simulink model "SolarPVMPPTBoost"  (R2025a)
settings: Solver=ode23t  StartTime=0.0  StopTime=t_sim2(end)  MaxStep=1/(10*solarPlant.converterSwitchingFrequency)  RelTol=1e-3  AbsTol=1e-3
PreLoadFcn:
  | run('SolarPVMPPTBoostData');
undefined symbols (not defined in the file or in its folder): boostController, dcVoltage, sensor, solarPanel, solarPlant
libraries: fl_lib x12, nesl_utility x10, simulink x6, ee_lib x3, batteryecm_lib x2, eePwmGenerator x2, simulink_extras x1
(part 1 of 2)
Description:
  | Solar PV System with MPPT Using Boost Converter
  | 
  | %
settings Model: Creator=The MathWorks, Inc.  LastModifiedBy=LaptopHP
settings SolverCC: AutoScaleAbsTol=off  AlgebraicLoopSolver=TrustRegion  MaxZcPerStep=1.0
settings DataIOCC: SaveOutput=off  DSMLogging=off  SaveTime=off  ReturnWorkspaceOutputs=off  SignalLoggingName=SolarPVMPPTBoost_logDB
settings OptimizationCC: ReuseModelBlockBuffer=off
settings DebuggingCC: UnconnectedInputMsg=warning  UnconnectedOutputMsg=warning  UnconnectedLineMsg=warning  SymbolicDimsDataTypeCodeGenerationDiagnostic=none
settings ModelReferenceCC: EnableRefExpFcnMdlSchedulingChecks=on
settings SFSimCC: CustomCodeUndefinedFunction=UseInterfaceOnly
settings RTWCC: GPUComputeCapability=3.5  DLArmComputeVersion=19.05
settings SimscapeCC: SimscapeLogType=all  SimscapeLogSimulationStatistics=on  SimscapeLogName=simlog_SolarPVMPPTBoost  SimscapeLogDataHistory=10000.0

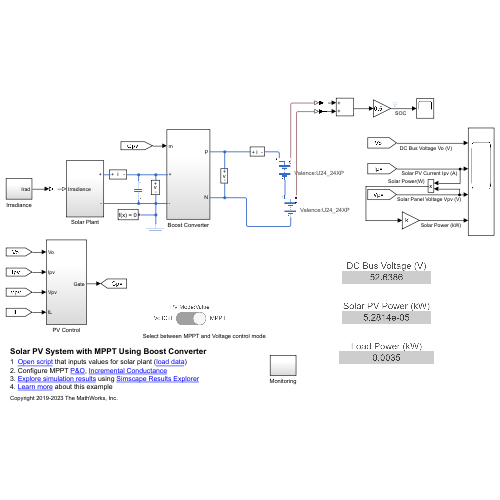
[thumbnail: Simulink's stored preview of the top-level diagram]
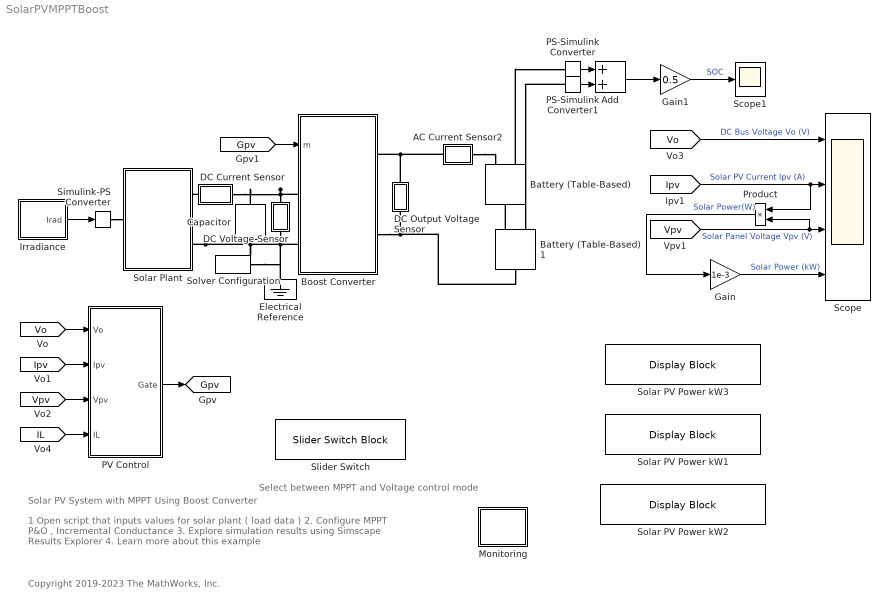
== system SolarPVMPPTBoost ==
  note: Select between MPPT and Voltage control mode
  note: Solar PV System with MPPT Using Boost Converter
  note: 1 Open script that inputs values for solar plant ( load data )
      | 2. Configure MPPT P&O , Incremental Conductance
      | 3. Explore simulation results using Simscape Results Explorer
      | 4. Learn more about this example
  note: Copyright 2019-2023 The MathWorks, Inc.
  AC Current Sensor2 : Subsystem
      mask Display: disp('i');
  Add : Sum
  Battery (Table-Based) : batteryecm_lib/Battery (Table-Based)  PartSpecification="{\"CollectionId\":\"SimscapeBatteryShared\",\"CollectionVersion\":\"1.0.0\",\"DatasetId\":\"Valence|U24_24XP|simscape.battery.batteryTableBased\",\"DisplayName\":\"Valence:U24_24XP\"}"  SOC_vec=[0 0.01 0.02 0.03 0.04 0.05 0.06 0.07 0.08 0.09 0.1 0.11 0.12 0.13 0.14 0.15 0.16 0.17 0.18 0.19 0.2 0.21 0.22 0.23 0.24 0.25 0.26 0.27 0.28 0.29 0.3 0.31 0.32 0.33 0.34 0.35 0.36 0.37 0.38 0.39 0.4 0.41 0.42 0.43 0.44 0.45 0.46 0.47 0.48 0.49 0.5 0.51 0.52 0.53 0.54 0.55 0.56 0.57 0.58 0.59 0.6 0.61 0.62 0.63 0.64 0.65 0.66 0.67 0.68 0.69 0.7 0.71 0.72 0.73 0.74 0.75 0.76 0.77 0.78 0.79 0.8 0.81 0.82 0.83 0.84 0.85 0.86 0.87 0.88 0.89 0.9 0.91 0.92 0.93 0.94 0.95 0.96 0.97 0.98 0.99 1] % Datasheet derived  T_dependence=simscape.enum.tablebattery.temperature_dependence.yes  prm_dir=simscape.enum.tablebattery.prm_dir.noCurrentDirectionality  T_vec=[-10 0 10 20 25 30 40 50] % Datasheet derived degC  V0_mat=[21.97161 21.97161 21.97161 21.97161 21.97161 21.97161 21.97161 21.97161;22.53804 22.53804 22.53804 22.53804 22.53804 22.53804 22.53804 22.53804;23.10446 23.10446 23.10446 23.10446 23.10446 23.10446 23.10446 23.10446;23.67089 23.67089 23.67089 23.67089 23.67089 23.67089 23.67089 23.67089;24.23731 24.23731 24.23731 24.23731 24.23731 24.23731 24.23731 24.23731;24.64924 24.64924 24.64924 24.64924 24.64924 24.64924 24.64924 24.64924;24.92163 24.92163 24.92163 24.92163 24.92163 24.92163 24.92163 24.92163;25.09504 25.09504 25.09504 25.09504 25.09504 25.09504 25.09504 25.09504;25.19187 25.19187 25.19187 25.19187 25.19187 25.19187 25.19187 25.19187;25.27387 25.27387 25.27387 25.27387 25.27387 25.27387 25.27387 25.27387;25.33805 25.33805 25.33805 25.33805 25.33805 25.33805 25.33805 25.33805;25.38759 25.38759 25.38759 25.38759 25.38759 25.38759 25.38759 25.38759;25.42722 25.42722 25.42722 25.42722 25.42722 25.42722 25.42722 25.42722;25.4595 25.4595 25.4595 25.4595 25.4595 25.4595 25.4595 25.4595;25.51339 25.51339 25.51339 25.51339 25.51339 25.51339 25.51339 25.51339;25.56513 25.56513 25.56513 25.56513 25.56513 25.56513 25.56513 25.56513;25.61607 25.61607 25.61607 25.61607 25.61607 25.61607 25.61607 25.61607;25.66568 25.66568 25.66568 25.66568 25.66568 25.66568 25.66568 25.66568;25.7036 25.7036 25.7036 25.7036 25.7036 25.7036 25.7036 25.7036;25.73844 25.73844 25.73844 25.73844 25.73844 25.73844 25.73844 25.73844;25.77746 25.77746 25.77746 25.77746 25.77746 25.77746 25.77746 25.77746;25.81538 25.81538 25.81538 25.81538 25.81538 25.81538 25.81538 25.81538;25.84852 25.84852 25.84852 25.84852 25.84852 25.84852 25.84852 25.84852;25.87416 25.87416 25.87416 25.87416 25.87416 25.87416 25.87416 25.87416;25.89973 25.89973 25.89973 25.89973 25.89973 25.89973 25.89973 25.89973;25.92218 25.92218 25.92218 25.92218 25.92218 25.92218 25.92218 25.92218;25.94447 25.94447 25.94447 25.94447 25.94447 25.94447 25.94447 25.94447;25.96638 25.96638 25.96638 25.96638 25.96638 25.96638 25.96638 25.96638;25.98898 25.98898 25.98898 25.98898 25.98898 25.98898 25.98898 25.98898;26.01189 26.01189 26.01189 26.01189 26.01189 26.01189 26.01189 26.01189;26.0314 26.0314 26.0314 26.0314 26.0314 26.0314 26.0314 26.0314;26.0479 26.0479 26.0479 26.0479 26.0479 26.0479 26.0479 26.0479;26.06442 26.06442 26.06442 26.06442 26.06442 26.06442 26.06442 26.06442;26.08147 26.08147 26.08147 26.08147 26.08147 26.08147 26.08147 26.08147;26.09966 26.09966 26.09966 26.09966 26.09966 26.09966 26.09966 26.09966;26.11433 26.11433 26.11433 26.11433 26.11433 26.11433 26.11433 26.11433;26.12673 26.12673 26.12673 26.12673 26.12673 26.12673 26.12673 26.12673;26.13904 26.13904 26.13904 26.13904 26.13904 26.13904 26.13904 26.13904;26.14842 26.14842 26.14842 26.14842 26.14842 26.14842 26.14842 26.14842;26.15721 26.15721 26.15721 26.15721 26.15721 26.15721 26.15721 26.15721;26.16347 26.16347 26.16347 26.16347 26.16347 26.16347 26.16347 26.16347;26.16814 26.16814 26.16814 26.16814 26.16814 26.16814 26.16814 26.16814;26.17307 26.17307 26.17307 26.17307 26.17307 26.17307 26.17307 26.17307;26.17807 26.17807 26.17807 26.17807 26.17807 26.17807 26.17807 26.17807;26.18238 26.18238 26.18238 26.18238 26.18238 26.18238 26.18238 26.18238;26.18632 26.18632 26.18632 26.18632 26.18632 26.18632 26.18632 26.18632;26.1904 26.1904 26.1904 26.1904 26.1904 26.1904 26.1904 26.1904;26.1947 26.1947 26.1947 26.1947 26.1947 26.1947 26.1947 26.1947;26.20065 26.20065 26.20065 26.20065 26.20065 26.20065 26.20065 26.20065;26.20672 26.20672 26.20672 26.20672 26.20672 26.20672 26.20672 26.20672;26.2124 26.2124 26.2124 26.2124 26.2124 26.2124 26.2124 26.2124;26.21806 26.21806 26.21806 26.21806 26.21806 26.21806 26.21806 26.21806;26.22346 26.22346 26.22346 26.22346 26.22346 26.22346 26.22346 26.22346;26.2281 26.2281 26.2281 26.2281 26.2281 26.2281 26.2281 26.2281;26.2334 26.2334 26.2334 26.2334 26.2334 26.2334 26.2334 26.2334;26.23938 26.23938 26.23938 26.23938 26.23938 26.23938 26.23938 26.23938;26.24642 26.24642 26.24642 26.24642 ...(+3164 chars)] % Datasheet derived V  V0_vec=[21.97161 22.53804 23.10446 23.67089 24.23731 24.64924 24.92163 25.09504 25.19187 25.27387 25.33805 25.38759 25.42722 25.4595 25.51339 25.56513 25.61607 25.66568 25.7036 25.73844 25.77746 25.81538 25.84852 25.87416 25.89973 25.92218 25.94447 25.96638 25.98898 26.01189 26.0314 26.0479 26.06442 26.08147 26.09966 26.11433 26.12673 26.13904 26.14842 26.15721 26.16347 26.16814 26.17307 26.17807 26.18238 26.18632 26.1904 26.1947 26.20065 26.20672 26.2124 26.21806 26.22346 26.2281 26.2334 26.23938 26.24642 26.25269 26.25896 26.26548 26.27379 26.2825 26.29069 26.30561 26.32142 26.33689 26.35375 26.37185 26.3921 26.41222 26.43078 26.44938 26.46076 26.47029 26.47968 26.48844 26.49691 26.50149 26.50599 26.51083 26.51604 26.52158 26.52717 26.53279 26.53633 26.53958 26.54323 26.54611 26.5485 26.55084 26.55294 26.5544 26.55643 26.55851 26.56043 26.5622 26.56188 26.56144 26.58586 26.70859 27.30705] % Datasheet derived V  V_range=[18 Inf] % Datasheet derived V  R0_mat=[0.54908 0.36314 0.2764 0.16088 0.05764 0.13571 0.12659 0.05774;0.54908 0.44265 0.26167 0.13798 0.05067 0.07244 0.03428 0.01604;0.54908 0.42379 0.24694 0.11508 0.04408 0.04315 0.01613 0.00642;0.54908 0.40494 0.23221 0.08791 0.03895 0.03189 0.01013 0.00208;0.54908 0.38608 0.21748 0.07667 0.03552 0.03066 0.00929 0.00422;0.54908 0.36723 0.19752 0.06478 0.03189 0.02569 0.01043 0.00535;0.54908 0.34837 0.17282 0.05789 0.02929 0.02227 0.00961 0.0053;0.53115 0.32952 0.14641 0.04918 0.02635 0.01969 0.00943 0.00609;0.51322 0.31066 0.12286 0.04116 0.02373 0.01811 0.01004 0.00662;0.4953 0.29181 0.10659 0.03522 0.02163 0.01754 0.01117 0.00795;0.47737 0.27295 0.08964 0.0314 0.01995 0.01744 0.01216 0.00949;0.45945 0.2541 0.07869 0.02828 0.01872 0.01722 0.01278 0.01054;0.44152 0.23524 0.0681 0.02622 0.01765 0.01699 0.01313 0.01128;0.42359 0.21639 0.05799 0.02448 0.01657 0.01661 0.01324 0.01172;0.40567 0.19753 0.05242 0.02411 0.01609 0.01701 0.01402 0.01221;0.38774 0.17868 0.04678 0.02358 0.0157 0.01718 0.01427 0.01246;0.36981 0.1579 0.04388 0.02288 0.0155 0.01718 0.01448 0.01249;0.35189 0.13912 0.0417 0.02324 0.01531 0.01733 0.01466 0.01266;0.33396 0.12244 0.03911 0.02318 0.01512 0.01719 0.01461 0.01278;0.31604 0.10756 0.037 0.02279 0.01496 0.01702 0.01461 0.01279;0.29811 0.09619 0.03588 0.0226 0.015 0.01715 0.01474 0.01297;0.28018 0.08561 0.03472 0.02261 0.01503 0.01735 0.01484 0.01311;0.26226 0.07746 0.03392 0.02245 0.01501 0.01748 0.015 0.01321;0.24433 0.07095 0.03328 0.02228 0.0149 0.01737 0.01498 0.01326;0.2264 0.06527 0.03264 0.02222 0.01484 0.01735 0.01496 0.01331;0.20848 0.06048 0.03189 0.02206 0.01484 0.01725 0.01484 0.01325;0.19055 0.05642 0.0314 0.02188 0.01483 0.01725 0.0148 0.0132;0.17261 0.05392 0.03124 0.02166 0.01482 0.01734 0.01474 0.01316;0.15623 0.05165 0.0311 0.0216 0.01484 0.01745 0.0147 0.01313;0.13985 0.05007 0.03098 0.02182 0.01488 0.01753 0.01467 0.01312;0.12469 0.04863 0.03074 0.02193 0.01488 0.01749 0.01458 0.01299;0.11172 0.04745 0.03039 0.02193 0.01485 0.01734 0.01441 0.01276;0.10133 0.04627 0.03021 0.02193 0.01482 0.0174 0.01423 0.01254;0.09285 0.04545 0.03014 0.02196 0.01481 0.01754 0.01408 0.01233;0.08571 0.04484 0.0301 0.02202 0.01486 0.01772 0.01421 0.01216;0.08062 0.04411 0.02994 0.02196 0.01488 0.01778 0.01442 0.01187;0.07546 0.04359 0.02971 0.02182 0.01488 0.01777 0.01455 0.0115;0.07174 0.04317 0.02947 0.02178 0.01489 0.01775 0.01468 0.01169;0.06901 0.04265 0.02927 0.02169 0.01486 0.01763 0.0147 0.0118;0.06625 0.04215 0.02911 0.02158 0.01483 0.01749 0.01468 0.01189;0.06412 0.04158 0.02886 0.02138 0.01477 0.01726 0.01453 0.01189;0.06209 0.04096 0.02856 0.02113 0.01469 0.01698 0.01434 0.01184;0.06059 0.04047 0.02827 0.02089 0.01463 0.01671 0.01415 0.0118;0.05926 0.04008 0.02798 0.02065 0.01457 0.01646 0.01396 0.01176;0.05791 0.03967 0.02766 0.02056 0.0145 0.01639 0.01394 0.0117;0.05724 0.03925 0.02734 0.02049 0.01443 0.01632 0.01391 0.01162;0.05657 0.03895 0.02718 0.02042 0.01436 0.01624 0.01389 0.01155;0.05592 0.0387 0.02709 0.02036 0.01429 0.01618 0.01387 0.01149;0.05535 0.0385 0.02705 0.02036 0.01425 0.01617 0.01391 0.01148;0.05481 0.0383 0.02702 0.02037 0.01422 0.01617 0.01388 0.01148;0.05426 0.03809 0.02697 0.02036 0.01417 0.01615 0.0138 0.01146;0.05371 0.03793 0.02693 0.02035 0.01413 0.01613 0.01372 0.01143;0.05347 0.0379 0.02688 0.02033 0.01408 0.01608 0.01363 0.0114;0.05325 0.03784 0.0268 0.02028 0.01402 0.01601 0.01351 0.01133;0.05305 0.03781 0.02674 0.02026 0.01397 0.01596 0.01342 0.01129;0.05287 0.03779 0.02671 0.0202 0.01394 0.01594 0.01335 0.01127;0.05282 0.03782 0.02671 0.02015 0.01396 0.01595 0.01334 0.01129;0.05295 0.03782 0.02669 0.02006 0.01397 0.01593 0.01335 0.01128;0.05307 0.03775 0.02667 0.01998 0.01398 0.01591 0.01337 0.01127;0.0532 0.03767 0.02665 0.01991 0.01399 0.01586 0.0134 0.01127;0.05339 0.03765 0.0267 0.0199 0.01403 0.01587 0.01349 0.01133;0.05359 0.03765 0.02676 0.0199 0.01406 0.01589 0.01359 0.01131;0.05376 0.03763 0.0268 0.0199 0.01407 0.0159 0.01365 0.01125;0.05415 0.03786 ...(+2366 chars)] % Datasheet derived Ohm  R0_vec=[0.05764 0.05067 0.04408 0.03895 0.03552 0.03189 0.02929 0.02635 0.02373 0.02163 0.01995 0.01872 0.01765 0.01657 0.01609 0.0157 0.0155 0.01531 0.01512 0.01496 0.015 0.01503 0.01501 0.0149 0.01484 0.01484 0.01483 0.01482 0.01484 0.01488 0.01488 0.01485 0.01482 0.01481 0.01486 0.01488 0.01488 0.01489 0.01486 0.01483 0.01477 0.01469 0.01463 0.01457 0.0145 0.01443 0.01436 0.01429 0.01425 0.01422 0.01417 0.01413 0.01408 0.01402 0.01397 0.01394 0.01396 0.01397 0.01398 0.01399 0.01403 0.01406 0.01407 0.01415 0.01424 0.01433 0.01444 0.01455 0.01469 0.01482 0.01493 0.01505 0.01508 0.01511 0.01513 0.01515 0.01517 0.01516 0.01514 0.01512 0.0151 0.0151 0.0151 0.01511 0.0151 0.01508 0.01507 0.01507 0.01507 0.01506 0.01504 0.01501 0.01495 0.0149 0.01485 0.01477 0.01458 0.01423 0.01378 0.01336 0.01453] % Datasheet derived Ohm  R0_dis_mat=[.0117, .0085, .009; .011, .0085, .009; .0114, .0087, .0092; .0107, .0082, .0088; .0107, .0083, .0091; .0113, .0085, .0089; .0116, .0085, .0089] % Parameter not set Ohm  R0_dis_vec=[.0085, .0085, .0087, .0082, .0083, .0085, .0085] % Parameter not set Ohm  R0_ch_mat=[.0117, .0085, .009; .011, .0085, .009; .0114, .0087, .0092; .0107, .0082, .0088; .0107, .0083, .0091; .0113, .0085, .0089; .0116, .0085, .0089] % Parameter not set Ohm  R0_ch_vec=[.0085, .0085, .0087, .0082, .0083, .0085, .0085] % Parameter not set Ohm  AH=0.002 hr*A  prm_leak=simscape.enum.tablebattery.prm_leak.disabled  Rleak_vec=[8000, 7000, 6000] % Parameter not set Ohm  Rleak=7e3 % Parameter not set Ohm  extrapolation_option=simscape.enum.extrapolation.nearest  SOC_port=simscape.enum.tablebattery.enable.yes  prm_dyn=simscape.enum.tablebattery.prm_dyn.off  R1_mat=[.0109, .0029, .0013; .0069, .0024, .0012; .0047, .0026, .0013; .0034, .0016, .001; .0033, .0023, .0014; .0033, .0018, .0011; .0028, .0017, .0011] % Parameter not set Ohm  R1_vec=[.0029, .0024, .0026, .0016, .0023, .0018, .0017] % Parameter not set Ohm  tau1_mat=[20, 36, 39; 31, 45, 39; 109, 105, 61; 36, 29, 26; 59, 77, 67; 40, 33, 29; 25, 39, 33] % Parameter not set s  tau1_vec=[36, 45, 105, 29, 77, 33, 39] % Parameter not set s  R2_mat=[.0109, .0029, .0013; .0069, .0024, .0012; .0047, .0026, .0013; .0034, .0016, .001; .0033, .0023, .0014; .0033, .0018, .0011; .0028, .0017, .0011] % Parameter not set Ohm  R2_vec=[.0029, .0024, .0026, .0016, .0023, .0018, .0017] % Parameter not set Ohm  tau2_mat=[20, 36, 39; 31, 45, 39; 109, 105, 61; 36, 29, 26; 59, 77, 67; 40, 33, 29; 25, 39, 33] % Parameter not set s  tau2_vec=[36, 45, 105, 29, 77, 33, 39] % Parameter not set s  R3_mat=[.0109, .0029, .0013; .0069, .0024, .0012; .0047, .0026, .0013; .0034, .0016, .001; .0033, .0023, .0014; .0033, .0018, .0011; .0028, .0017, .0011] % Parameter not set Ohm  R3_vec=[.0029, .0024, .0026, .0016, .0023, .0018, .0017] % Parameter not set Ohm  tau3_mat=[20, 36, 39; 31, 45, 39; 109, 105, 61; 36, 29, 26; 59, 77, 67; 40, 33, 29; 25, 39, 33] % Parameter not set s  tau3_vec=[36, 45, 105, 29, 77, 33, 39] % Parameter not set s  R4_mat=[.0109, .0029, .0013; .0069, .0024, .0012; .0047, .0026, .0013; .0034, .0016, .001; .0033, .0023, .0014; .0033, .0018, .0011; .0028, .0017, .0011] % Parameter not set Ohm  R4_vec=[.0029, .0024, .0026, .0016, .0023, .0018, .0017] % Parameter not set Ohm  tau4_mat=[20, 36, 39; 31, 45, 39; 109, 105, 61; 36, 29, 26; 59, 77, 67; 40, 33, 29; 25, 39, 33] % Parameter not set s  tau4_vec=[36, 45, 105, 29, 77, 33, 39] % Parameter not set s  R5_mat=[.0109, .0029, .0013; .0069, .0024, .0012; .0047, .0026, .0013; .0034, .0016, .001; .0033, .0023, .0014; .0033, .0018, .0011; .0028, .0017, .0011] % Parameter not set Ohm  R5_vec=[.0029, .0024, .0026, .0016, .0023, .0018, .0017] % Parameter not set Ohm  tau5_mat=[20, 36, 39; 31, 45, 39; 109, 105, 61; 36, 29, 26; 59, 77, 67; 40, 33, 29; 25, 39, 33] % Parameter not set s  tau5_vec=[36, 45, 105, 29, 77, 33, 39] % Parameter not set s  prm_fade=simscape.enum.tablebattery.prm_fade.tableN  N0=100 % Parameter not set  dV0=0 % Parameter not set  dR0=0 % Parameter not set  dAH=0 % Parameter not set  dRleak=0 % Parameter not set  dR1=0 % Parameter not set  dR2=0 % Parameter not set  dR3=0 % Parameter not set  dR4=0 % Parameter not set  dR5=0 % Parameter not set  N0vec=[0 49 97 145 193 241 289 337 385 433 481 529 577 625 673 721 769 817 865 913 961 1009 1057 1105 1153 1201 1249 1297 1345 1393 1441 1489 1537 1585 1633 1681 1729 1777 1825 1873 1921 1969 2017 2065 2113 2161 2209 2257 2305 2353 2401 2449 2497 2545 2593 2641 2689 2737 2785 2833 2881 2929 2977 3025 3073 3121 3169 3217 3265 3313 3361 3409 3457 3505 3553 3601 3649 3697 3745 3793 3841 3889 3937 3985 4033 4081 4129 4177 4225 4273 4321 4369 4417 4465 4513 4561 4609 4657 4705 4753] % Datasheet derived  Tfadevec=[298.15, 323.15] % Parameter not set K  dV0vec=[0 -1.0347 -2.0695 -2.3787 -2.5909 -2.6684 -2.7051 -2.7303 -2.7296 -2.7289 -2.7284 -2.728 -2.7283 -2.7308 -2.7333 -2.7359 -2.7386 -2.741 -2.7436 -2.7462 -2.7488 -2.7513 -2.7539 -2.7564 -2.7587 -2.7612 -2.7646 -2.7682 -2.772 -2.776 -2.7801 -2.7841 -2.7877 -2.7918 -2.7958 -2.8006 -2.8058 -2.8109 -2.8155 -2.8205 -2.8258 -2.8314 -2.8378 -2.8465 -2.8557 -2.8649 -2.8742 -2.8834 -2.8925 -2.9014 -2.91 -2.9189 -2.9284 -2.9375 -2.9463 -2.9552 -2.9641 -2.9784 -2.995 -3.012 -3.0272 -3.0424 -3.0579 -3.0735 -3.0893 -3.1061 -3.1249 -3.1454 -3.1761 -3.2068 -3.2374 -3.268 -3.3004 -3.3401 -3.381 -3.4219 -3.4587 -3.495 -3.529 -3.5622 -3.5934 -3.625 -3.6559 -3.6845 -3.7125 -3.7321 -3.7475 -3.7635 -3.7799 -3.7956 -3.8112 -3.8287 -3.8469 -3.8647 -3.8826 -3.9025 -3.9206 -3.937 -3.9519 -3.9651] % Datasheet derived  dR0vec=[0 0 0 0 0 0 0 0 0 0 0 0 0 0 0 0 0 0 0 0 0 0 0 0 0 0 0 0 0 0 0 0 0 0 0 0 0 0 0 0 0 0 0 0 0 0 0 0 0 0 0 0 0 0 0 0 0 0 0 0 0 0 0 0 0 0 0 0 0 0 0 0 0 0 0 0 0 0 0 0 0 0 0 0 0 0 0 0 0 0 0 0 0 0 0 0 0 0 0 0] % Parameter assumed  dAHvec=[0 -0.472 -0.944 -1.416 -1.889 -2.306 -2.716 -3.125 -3.535 -3.944 -4.342 -4.723 -5.104 -5.485 -5.867 -6.248 -6.629 -6.972 -7.314 -7.656 -7.997 -8.339 -8.681 -9.022 -9.457 -9.923 -10.389 -10.855 -11.321 -11.787 -12.254 -12.72 -13.106 -13.491 -13.876 -14.262 -14.647 -15.032 -15.417 -15.837 -16.264 -16.69 -17.116 -17.542 -17.987 -18.438 -18.889 -19.341 -19.792 -20.243 -20.694 -21.177 -21.71 -22.243 -22.776 -23.309 -23.842 -24.376 -24.909 -25.442 -25.915 -26.366 -26.816 -27.266 -27.717 -28.167 -28.617 -29.068 -29.518 -29.968 -30.419 -30.869 -31.319 -31.858 -32.41 -32.961 -33.512 -34.063 -34.615 -35.166 -35.717 -36.269 -36.802 -37.314 -37.826 -38.339 -38.851 -39.363 -39.875 -40.388 -40.9 -41.603 -42.38 -43.158 -43.935 -44.712 -45.49 -46.267 -47.044 -47.822] % Datasheet derived  dRleakvec=[0, 0, 0, 0] % Parameter not set  dR1vec=[0, 0, 0, 0] % Parameter not set  dR2vec=[0, 0, 0, 0] % Parameter not set  dR3vec=[0, 0, 0, 0] % Parameter not set  dR4vec=[0, 0, 0, 0] % Parameter not set  dR5vec=[0, 0, 0, 0] % Parameter not set  dV0mat=[0, 0; 0, 0; 0, 0; 0, 0] % Parameter not set  dR0mat=[0, 0; 0, 0; 0, 0; 0, 0] % Parameter not set  dAHmat=[0, 0; 0, 0; 0, 0; 0, 0] % Parameter not set  dRleakmat=[0, 0; 0, 0; 0, 0; 0, 0] % Parameter not set  dR1mat=[0, 0; 0, 0; 0, 0; 0, 0] % Parameter not set  dR2mat=[0, 0; 0, 0; 0, 0; 0, 0] % Parameter not set  dR3mat=[0, 0; 0, 0; 0, 0; 0, 0] % Parameter not set  dR4mat=[0, 0; 0, 0; 0, 0; 0, 0] % Parameter not set  dR5mat=[0, 0; 0, 0; 0, 0; 0, 0] % Parameter not set  prm_age_modeling=simscape.enum.tablebattery.prm_age_modeling.equation  storage_dt_age_vec=[0] % Parameter not set d  storage_T_age_vec=[273] % Parameter not set K  prm_age_OCV=simscape.enum.tablebattery.prm_age_OCV.OCV  OCV_age=0.9 % Parameter not set  SOC_age=0.6 % Parameter not set  prm_age_resistance=simscape.enum.tablebattery.prm_age.disabled  OCV_scaling_age_resistance=2.2134e6 % Parameter not set  OCV_offset_age_resistance=1.632e6 % Parameter not set  temp_exp_age_resistance=0.515833569 % Parameter not set V  t_exp_age_resistance=0.75 % Parameter not set  T_age_vec_resistance=[273.15, 298.15, 323.15] % Parameter not set K  dt_age_vec_resistance=[0, 90, 180, 270] % Parameter not set d  dR0_age_vec=[0, 0, 0] % Parameter not set  t_meas_dR0_age=100 % Parameter not set d  dR0_age_mat=[0, 0, 0; 0, 0, 0; 0, 0, 0; 0, 0, 0] % Parameter not set  prm_age_capacity=simscape.enum.tablebattery.prm_age.disabled  OCV_scaling_age_capacity=1.5097e07 % Parameter not set  OCV_offset_age_capacity=8.3625e06 % Parameter not set  temp_exp_age_capacity=0.6011 % Parameter not set V  t_exp_age_capacity=0.75 % Parameter not set  T_age_vec_capacity=[273.15, 298.15, 323.15] % Parameter not set K  dt_age_vec_capacity=[0, 90, 180, 270] % Parameter not set d  dAH_age_vec=[0, 0, 0] % Parameter not set  t_meas_dAH_age=100 % Parameter not set d  dAH_age_mat=[0, 0, 0; 0, 0, 0; 0, 0, 0; 0, 0, 0] % Parameter not set  thermal_port=simscape.enum.thermaleffects.omit  temperature=298.15 % Parameter not set K  thermal_mass=14670 % Parameter assumed J/K  i_specify=off  i_priority=None  i=0 A  i_nominal_specify=off  i_nominal_value=1  i_nominal_unit=A  v_specify=off  v_priority=None  v=0 V  v_nominal_specify=off  v_nominal_value=1  v_nominal_unit=V  stateOfCharge_specify=on  stateOfCharge_priority=High  stateOfCharge=0.2  stateOfCharge_nominal_specify=off  stateOfCharge_nominal_value=1  stateOfCharge_nominal_unit=1  num_cycles_specify=off  num_cycles_priority=High  num_cycles=0  num_cycles_nominal_specify=off  num_cycles_nominal_value=1  num_cycles_nominal_unit=1  cell_temperature_specify=off  cell_temperature_priority=High  cell_temperature=298.15 K  cell_temperature_nominal_specify=off  cell_temperature_nominal_value=1  cell_temperature_nominal_unit=K
      settings: AttributesFormatString=Valence:U24_24XP  InternalSimscapePortConfiguration="{\"Bottom\":[],\"Left\":[{\"id\":\"p\",\"label\":\"+\",\"type\":\"foundation.electrical.electrical\"},{\"id\":\"soc\",\"label\":\"SOC\",\"type\":\"output\"}],\"Right\":[{\"id\":\"n\",\"label\":\"-\",\"type\":\"foundation.electrical.electrical\"}],\"Top\":[]}"
      settings: LibrarySourceBlock=|
      | batt_lib/Cells/Battery
      | (Table-Based)
  Battery (Table-Based)1 : batteryecm_lib/Battery (Table-Based)  PartSpecification="{\"CollectionId\":\"SimscapeBatteryShared\",\"CollectionVersion\":\"1.0.0\",\"DatasetId\":\"Valence|U24_24XP|simscape.battery.batteryTableBased\",\"DisplayName\":\"Valence:U24_24XP\"}"  SOC_vec=[0 0.01 0.02 0.03 0.04 0.05 0.06 0.07 0.08 0.09 0.1 0.11 0.12 0.13 0.14 0.15 0.16 0.17 0.18 0.19 0.2 0.21 0.22 0.23 0.24 0.25 0.26 0.27 0.28 0.29 0.3 0.31 0.32 0.33 0.34 0.35 0.36 0.37 0.38 0.39 0.4 0.41 0.42 0.43 0.44 0.45 0.46 0.47 0.48 0.49 0.5 0.51 0.52 0.53 0.54 0.55 0.56 0.57 0.58 0.59 0.6 0.61 0.62 0.63 0.64 0.65 0.66 0.67 0.68 0.69 0.7 0.71 0.72 0.73 0.74 0.75 0.76 0.77 0.78 0.79 0.8 0.81 0.82 0.83 0.84 0.85 0.86 0.87 0.88 0.89 0.9 0.91 0.92 0.93 0.94 0.95 0.96 0.97 0.98 0.99 1] % Datasheet derived  T_dependence=simscape.enum.tablebattery.temperature_dependence.yes  prm_dir=simscape.enum.tablebattery.prm_dir.noCurrentDirectionality  T_vec=[-10 0 10 20 25 30 40 50] % Datasheet derived degC  V0_mat=[21.97161 21.97161 21.97161 21.97161 21.97161 21.97161 21.97161 21.97161;22.53804 22.53804 22.53804 22.53804 22.53804 22.53804 22.53804 22.53804;23.10446 23.10446 23.10446 23.10446 23.10446 23.10446 23.10446 23.10446;23.67089 23.67089 23.67089 23.67089 23.67089 23.67089 23.67089 23.67089;24.23731 24.23731 24.23731 24.23731 24.23731 24.23731 24.23731 24.23731;24.64924 24.64924 24.64924 24.64924 24.64924 24.64924 24.64924 24.64924;24.92163 24.92163 24.92163 24.92163 24.92163 24.92163 24.92163 24.92163;25.09504 25.09504 25.09504 25.09504 25.09504 25.09504 25.09504 25.09504;25.19187 25.19187 25.19187 25.19187 25.19187 25.19187 25.19187 25.19187;25.27387 25.27387 25.27387 25.27387 25.27387 25.27387 25.27387 25.27387;25.33805 25.33805 25.33805 25.33805 25.33805 25.33805 25.33805 25.33805;25.38759 25.38759 25.38759 25.38759 25.38759 25.38759 25.38759 25.38759;25.42722 25.42722 25.42722 25.42722 25.42722 25.42722 25.42722 25.42722;25.4595 25.4595 25.4595 25.4595 25.4595 25.4595 25.4595 25.4595;25.51339 25.51339 25.51339 25.51339 25.51339 25.51339 25.51339 25.51339;25.56513 25.56513 25.56513 25.56513 25.56513 25.56513 25.56513 25.56513;25.61607 25.61607 25.61607 25.61607 25.61607 25.61607 25.61607 25.61607;25.66568 25.66568 25.66568 25.66568 25.66568 25.66568 25.66568 25.66568;25.7036 25.7036 25.7036 25.7036 25.7036 25.7036 25.7036 25.7036;25.73844 25.73844 25.73844 25.73844 25.73844 25.73844 25.73844 25.73844;25.77746 25.77746 25.77746 25.77746 25.77746 25.77746 25.77746 25.77746;25.81538 25.81538 25.81538 25.81538 25.81538 25.81538 25.81538 25.81538;25.84852 25.84852 25.84852 25.84852 25.84852 25.84852 25.84852 25.84852;25.87416 25.87416 25.87416 25.87416 25.87416 25.87416 25.87416 25.87416;25.89973 25.89973 25.89973 25.89973 25.89973 25.89973 25.89973 25.89973;25.92218 25.92218 25.92218 25.92218 25.92218 25.92218 25.92218 25.92218;25.94447 25.94447 25.94447 25.94447 25.94447 25.94447 25.94447 25.94447;25.96638 25.96638 25.96638 25.96638 25.96638 25.96638 25.96638 25.96638;25.98898 25.98898 25.98898 25.98898 25.98898 25.98898 25.98898 25.98898;26.01189 26.01189 26.01189 26.01189 26.01189 26.01189 26.01189 26.01189;26.0314 26.0314 26.0314 26.0314 26.0314 26.0314 26.0314 26.0314;26.0479 26.0479 26.0479 26.0479 26.0479 26.0479 26.0479 26.0479;26.06442 26.06442 26.06442 26.06442 26.06442 26.06442 26.06442 26.06442;26.08147 26.08147 26.08147 26.08147 26.08147 26.08147 26.08147 26.08147;26.09966 26.09966 26.09966 26.09966 26.09966 26.09966 26.09966 26.09966;26.11433 26.11433 26.11433 26.11433 26.11433 26.11433 26.11433 26.11433;26.12673 26.12673 26.12673 26.12673 26.12673 26.12673 26.12673 26.12673;26.13904 26.13904 26.13904 26.13904 26.13904 26.13904 26.13904 26.13904;26.14842 26.14842 26.14842 26.14842 26.14842 26.14842 26.14842 26.14842;26.15721 26.15721 26.15721 26.15721 26.15721 26.15721 26.15721 26.15721;26.16347 26.16347 26.16347 26.16347 26.16347 26.16347 26.16347 26.16347;26.16814 26.16814 26.16814 26.16814 26.16814 26.16814 26.16814 26.16814;26.17307 26.17307 26.17307 26.17307 26.17307 26.17307 26.17307 26.17307;26.17807 26.17807 26.17807 26.17807 26.17807 26.17807 26.17807 26.17807;26.18238 26.18238 26.18238 26.18238 26.18238 26.18238 26.18238 26.18238;26.18632 26.18632 26.18632 26.18632 26.18632 26.18632 26.18632 26.18632;26.1904 26.1904 26.1904 26.1904 26.1904 26.1904 26.1904 26.1904;26.1947 26.1947 26.1947 26.1947 26.1947 26.1947 26.1947 26.1947;26.20065 26.20065 26.20065 26.20065 26.20065 26.20065 26.20065 26.20065;26.20672 26.20672 26.20672 26.20672 26.20672 26.20672 26.20672 26.20672;26.2124 26.2124 26.2124 26.2124 26.2124 26.2124 26.2124 26.2124;26.21806 26.21806 26.21806 26.21806 26.21806 26.21806 26.21806 26.21806;26.22346 26.22346 26.22346 26.22346 26.22346 26.22346 26.22346 26.22346;26.2281 26.2281 26.2281 26.2281 26.2281 26.2281 26.2281 26.2281;26.2334 26.2334 26.2334 26.2334 26.2334 26.2334 26.2334 26.2334;26.23938 26.23938 26.23938 26.23938 26.23938 26.23938 26.23938 26.23938;26.24642 26.24642 26.24642 26.24642 ...(+3164 chars)] % Datasheet derived V  V0_vec=[21.97161 22.53804 23.10446 23.67089 24.23731 24.64924 24.92163 25.09504 25.19187 25.27387 25.33805 25.38759 25.42722 25.4595 25.51339 25.56513 25.61607 25.66568 25.7036 25.73844 25.77746 25.81538 25.84852 25.87416 25.89973 25.92218 25.94447 25.96638 25.98898 26.01189 26.0314 26.0479 26.06442 26.08147 26.09966 26.11433 26.12673 26.13904 26.14842 26.15721 26.16347 26.16814 26.17307 26.17807 26.18238 26.18632 26.1904 26.1947 26.20065 26.20672 26.2124 26.21806 26.22346 26.2281 26.2334 26.23938 26.24642 26.25269 26.25896 26.26548 26.27379 26.2825 26.29069 26.30561 26.32142 26.33689 26.35375 26.37185 26.3921 26.41222 26.43078 26.44938 26.46076 26.47029 26.47968 26.48844 26.49691 26.50149 26.50599 26.51083 26.51604 26.52158 26.52717 26.53279 26.53633 26.53958 26.54323 26.54611 26.5485 26.55084 26.55294 26.5544 26.55643 26.55851 26.56043 26.5622 26.56188 26.56144 26.58586 26.70859 27.30705] % Datasheet derived V  V_range=[18 Inf] % Datasheet derived V  R0_mat=[0.54908 0.36314 0.2764 0.16088 0.05764 0.13571 0.12659 0.05774;0.54908 0.44265 0.26167 0.13798 0.05067 0.07244 0.03428 0.01604;0.54908 0.42379 0.24694 0.11508 0.04408 0.04315 0.01613 0.00642;0.54908 0.40494 0.23221 0.08791 0.03895 0.03189 0.01013 0.00208;0.54908 0.38608 0.21748 0.07667 0.03552 0.03066 0.00929 0.00422;0.54908 0.36723 0.19752 0.06478 0.03189 0.02569 0.01043 0.00535;0.54908 0.34837 0.17282 0.05789 0.02929 0.02227 0.00961 0.0053;0.53115 0.32952 0.14641 0.04918 0.02635 0.01969 0.00943 0.00609;0.51322 0.31066 0.12286 0.04116 0.02373 0.01811 0.01004 0.00662;0.4953 0.29181 0.10659 0.03522 0.02163 0.01754 0.01117 0.00795;0.47737 0.27295 0.08964 0.0314 0.01995 0.01744 0.01216 0.00949;0.45945 0.2541 0.07869 0.02828 0.01872 0.01722 0.01278 0.01054;0.44152 0.23524 0.0681 0.02622 0.01765 0.01699 0.01313 0.01128;0.42359 0.21639 0.05799 0.02448 0.01657 0.01661 0.01324 0.01172;0.40567 0.19753 0.05242 0.02411 0.01609 0.01701 0.01402 0.01221;0.38774 0.17868 0.04678 0.02358 0.0157 0.01718 0.01427 0.01246;0.36981 0.1579 0.04388 0.02288 0.0155 0.01718 0.01448 0.01249;0.35189 0.13912 0.0417 0.02324 0.01531 0.01733 0.01466 0.01266;0.33396 0.12244 0.03911 0.02318 0.01512 0.01719 0.01461 0.01278;0.31604 0.10756 0.037 0.02279 0.01496 0.01702 0.01461 0.01279;0.29811 0.09619 0.03588 0.0226 0.015 0.01715 0.01474 0.01297;0.28018 0.08561 0.03472 0.02261 0.01503 0.01735 0.01484 0.01311;0.26226 0.07746 0.03392 0.02245 0.01501 0.01748 0.015 0.01321;0.24433 0.07095 0.03328 0.02228 0.0149 0.01737 0.01498 0.01326;0.2264 0.06527 0.03264 0.02222 0.01484 0.01735 0.01496 0.01331;0.20848 0.06048 0.03189 0.02206 0.01484 0.01725 0.01484 0.01325;0.19055 0.05642 0.0314 0.02188 0.01483 0.01725 0.0148 0.0132;0.17261 0.05392 0.03124 0.02166 0.01482 0.01734 0.01474 0.01316;0.15623 0.05165 0.0311 0.0216 0.01484 0.01745 0.0147 0.01313;0.13985 0.05007 0.03098 0.02182 0.01488 0.01753 0.01467 0.01312;0.12469 0.04863 0.03074 0.02193 0.01488 0.01749 0.01458 0.01299;0.11172 0.04745 0.03039 0.02193 0.01485 0.01734 0.01441 0.01276;0.10133 0.04627 0.03021 0.02193 0.01482 0.0174 0.01423 0.01254;0.09285 0.04545 0.03014 0.02196 0.01481 0.01754 0.01408 0.01233;0.08571 0.04484 0.0301 0.02202 0.01486 0.01772 0.01421 0.01216;0.08062 0.04411 0.02994 0.02196 0.01488 0.01778 0.01442 0.01187;0.07546 0.04359 0.02971 0.02182 0.01488 0.01777 0.01455 0.0115;0.07174 0.04317 0.02947 0.02178 0.01489 0.01775 0.01468 0.01169;0.06901 0.04265 0.02927 0.02169 0.01486 0.01763 0.0147 0.0118;0.06625 0.04215 0.02911 0.02158 0.01483 0.01749 0.01468 0.01189;0.06412 0.04158 0.02886 0.02138 0.01477 0.01726 0.01453 0.01189;0.06209 0.04096 0.02856 0.02113 0.01469 0.01698 0.01434 0.01184;0.06059 0.04047 0.02827 0.02089 0.01463 0.01671 0.01415 0.0118;0.05926 0.04008 0.02798 0.02065 0.01457 0.01646 0.01396 0.01176;0.05791 0.03967 0.02766 0.02056 0.0145 0.01639 0.01394 0.0117;0.05724 0.03925 0.02734 0.02049 0.01443 0.01632 0.01391 0.01162;0.05657 0.03895 0.02718 0.02042 0.01436 0.01624 0.01389 0.01155;0.05592 0.0387 0.02709 0.02036 0.01429 0.01618 0.01387 0.01149;0.05535 0.0385 0.02705 0.02036 0.01425 0.01617 0.01391 0.01148;0.05481 0.0383 0.02702 0.02037 0.01422 0.01617 0.01388 0.01148;0.05426 0.03809 0.02697 0.02036 0.01417 0.01615 0.0138 0.01146;0.05371 0.03793 0.02693 0.02035 0.01413 0.01613 0.01372 0.01143;0.05347 0.0379 0.02688 0.02033 0.01408 0.01608 0.01363 0.0114;0.05325 0.03784 0.0268 0.02028 0.01402 0.01601 0.01351 0.01133;0.05305 0.03781 0.02674 0.02026 0.01397 0.01596 0.01342 0.01129;0.05287 0.03779 0.02671 0.0202 0.01394 0.01594 0.01335 0.01127;0.05282 0.03782 0.02671 0.02015 0.01396 0.01595 0.01334 0.01129;0.05295 0.03782 0.02669 0.02006 0.01397 0.01593 0.01335 0.01128;0.05307 0.03775 0.02667 0.01998 0.01398 0.01591 0.01337 0.01127;0.0532 0.03767 0.02665 0.01991 0.01399 0.01586 0.0134 0.01127;0.05339 0.03765 0.0267 0.0199 0.01403 0.01587 0.01349 0.01133;0.05359 0.03765 0.02676 0.0199 0.01406 0.01589 0.01359 0.01131;0.05376 0.03763 0.0268 0.0199 0.01407 0.0159 0.01365 0.01125;0.05415 0.03786 ...(+2366 chars)] % Datasheet derived Ohm  R0_vec=[0.05764 0.05067 0.04408 0.03895 0.03552 0.03189 0.02929 0.02635 0.02373 0.02163 0.01995 0.01872 0.01765 0.01657 0.01609 0.0157 0.0155 0.01531 0.01512 0.01496 0.015 0.01503 0.01501 0.0149 0.01484 0.01484 0.01483 0.01482 0.01484 0.01488 0.01488 0.01485 0.01482 0.01481 0.01486 0.01488 0.01488 0.01489 0.01486 0.01483 0.01477 0.01469 0.01463 0.01457 0.0145 0.01443 0.01436 0.01429 0.01425 0.01422 0.01417 0.01413 0.01408 0.01402 0.01397 0.01394 0.01396 0.01397 0.01398 0.01399 0.01403 0.01406 0.01407 0.01415 0.01424 0.01433 0.01444 0.01455 0.01469 0.01482 0.01493 0.01505 0.01508 0.01511 0.01513 0.01515 0.01517 0.01516 0.01514 0.01512 0.0151 0.0151 0.0151 0.01511 0.0151 0.01508 0.01507 0.01507 0.01507 0.01506 0.01504 0.01501 0.01495 0.0149 0.01485 0.01477 0.01458 0.01423 0.01378 0.01336 0.01453] % Datasheet derived Ohm  R0_dis_mat=[.0117, .0085, .009; .011, .0085, .009; .0114, .0087, .0092; .0107, .0082, .0088; .0107, .0083, .0091; .0113, .0085, .0089; .0116, .0085, .0089] % Parameter not set Ohm  R0_dis_vec=[.0085, .0085, .0087, .0082, .0083, .0085, .0085] % Parameter not set Ohm  R0_ch_mat=[.0117, .0085, .009; .011, .0085, .009; .0114, .0087, .0092; .0107, .0082, .0088; .0107, .0083, .0091; .0113, .0085, .0089; .0116, .0085, .0089] % Parameter not set Ohm  R0_ch_vec=[.0085, .0085, .0087, .0082, .0083, .0085, .0085] % Parameter not set Ohm  AH=0.002 hr*A  prm_leak=simscape.enum.tablebattery.prm_leak.disabled  Rleak_vec=[8000, 7000, 6000] % Parameter not set Ohm  Rleak=7e3 % Parameter not set Ohm  extrapolation_option=simscape.enum.extrapolation.nearest  SOC_port=simscape.enum.tablebattery.enable.yes  prm_dyn=simscape.enum.tablebattery.prm_dyn.off  R1_mat=[.0109, .0029, .0013; .0069, .0024, .0012; .0047, .0026, .0013; .0034, .0016, .001; .0033, .0023, .0014; .0033, .0018, .0011; .0028, .0017, .0011] % Parameter not set Ohm  R1_vec=[.0029, .0024, .0026, .0016, .0023, .0018, .0017] % Parameter not set Ohm  tau1_mat=[20, 36, 39; 31, 45, 39; 109, 105, 61; 36, 29, 26; 59, 77, 67; 40, 33, 29; 25, 39, 33] % Parameter not set s  tau1_vec=[36, 45, 105, 29, 77, 33, 39] % Parameter not set s  R2_mat=[.0109, .0029, .0013; .0069, .0024, .0012; .0047, .0026, .0013; .0034, .0016, .001; .0033, .0023, .0014; .0033, .0018, .0011; .0028, .0017, .0011] % Parameter not set Ohm  R2_vec=[.0029, .0024, .0026, .0016, .0023, .0018, .0017] % Parameter not set Ohm  tau2_mat=[20, 36, 39; 31, 45, 39; 109, 105, 61; 36, 29, 26; 59, 77, 67; 40, 33, 29; 25, 39, 33] % Parameter not set s  tau2_vec=[36, 45, 105, 29, 77, 33, 39] % Parameter not set s  R3_mat=[.0109, .0029, .0013; .0069, .0024, .0012; .0047, .0026, .0013; .0034, .0016, .001; .0033, .0023, .0014; .0033, .0018, .0011; .0028, .0017, .0011] % Parameter not set Ohm  R3_vec=[.0029, .0024, .0026, .0016, .0023, .0018, .0017] % Parameter not set Ohm  tau3_mat=[20, 36, 39; 31, 45, 39; 109, 105, 61; 36, 29, 26; 59, 77, 67; 40, 33, 29; 25, 39, 33] % Parameter not set s  tau3_vec=[36, 45, 105, 29, 77, 33, 39] % Parameter not set s  R4_mat=[.0109, .0029, .0013; .0069, .0024, .0012; .0047, .0026, .0013; .0034, .0016, .001; .0033, .0023, .0014; .0033, .0018, .0011; .0028, .0017, .0011] % Parameter not set Ohm  R4_vec=[.0029, .0024, .0026, .0016, .0023, .0018, .0017] % Parameter not set Ohm  tau4_mat=[20, 36, 39; 31, 45, 39; 109, 105, 61; 36, 29, 26; 59, 77, 67; 40, 33, 29; 25, 39, 33] % Parameter not set s  tau4_vec=[36, 45, 105, 29, 77, 33, 39] % Parameter not set s  R5_mat=[.0109, .0029, .0013; .0069, .0024, .0012; .0047, .0026, .0013; .0034, .0016, .001; .0033, .0023, .0014; .0033, .0018, .0011; .0028, .0017, .0011] % Parameter not set Ohm  R5_vec=[.0029, .0024, .0026, .0016, .0023, .0018, .0017] % Parameter not set Ohm  tau5_mat=[20, 36, 39; 31, 45, 39; 109, 105, 61; 36, 29, 26; 59, 77, 67; 40, 33, 29; 25, 39, 33] % Parameter not set s  tau5_vec=[36, 45, 105, 29, 77, 33, 39] % Parameter not set s  prm_fade=simscape.enum.tablebattery.prm_fade.tableN  N0=100 % Parameter not set  dV0=0 % Parameter not set  dR0=0 % Parameter not set  dAH=0 % Parameter not set  dRleak=0 % Parameter not set  dR1=0 % Parameter not set  dR2=0 % Parameter not set  dR3=0 % Parameter not set  dR4=0 % Parameter not set  dR5=0 % Parameter not set  N0vec=[0 49 97 145 193 241 289 337 385 433 481 529 577 625 673 721 769 817 865 913 961 1009 1057 1105 1153 1201 1249 1297 1345 1393 1441 1489 1537 1585 1633 1681 1729 1777 1825 1873 1921 1969 2017 2065 2113 2161 2209 2257 2305 2353 2401 2449 2497 2545 2593 2641 2689 2737 2785 2833 2881 2929 2977 3025 3073 3121 3169 3217 3265 3313 3361 3409 3457 3505 3553 3601 3649 3697 3745 3793 3841 3889 3937 3985 4033 4081 4129 4177 4225 4273 4321 4369 4417 4465 4513 4561 4609 4657 4705 4753] % Datasheet derived  Tfadevec=[298.15, 323.15] % Parameter not set K  dV0vec=[0 -1.0347 -2.0695 -2.3787 -2.5909 -2.6684 -2.7051 -2.7303 -2.7296 -2.7289 -2.7284 -2.728 -2.7283 -2.7308 -2.7333 -2.7359 -2.7386 -2.741 -2.7436 -2.7462 -2.7488 -2.7513 -2.7539 -2.7564 -2.7587 -2.7612 -2.7646 -2.7682 -2.772 -2.776 -2.7801 -2.7841 -2.7877 -2.7918 -2.7958 -2.8006 -2.8058 -2.8109 -2.8155 -2.8205 -2.8258 -2.8314 -2.8378 -2.8465 -2.8557 -2.8649 -2.8742 -2.8834 -2.8925 -2.9014 -2.91 -2.9189 -2.9284 -2.9375 -2.9463 -2.9552 -2.9641 -2.9784 -2.995 -3.012 -3.0272 -3.0424 -3.0579 -3.0735 -3.0893 -3.1061 -3.1249 -3.1454 -3.1761 -3.2068 -3.2374 -3.268 -3.3004 -3.3401 -3.381 -3.4219 -3.4587 -3.495 -3.529 -3.5622 -3.5934 -3.625 -3.6559 -3.6845 -3.7125 -3.7321 -3.7475 -3.7635 -3.7799 -3.7956 -3.8112 -3.8287 -3.8469 -3.8647 -3.8826 -3.9025 -3.9206 -3.937 -3.9519 -3.9651] % Datasheet derived  dR0vec=[0 0 0 0 0 0 0 0 0 0 0 0 0 0 0 0 0 0 0 0 0 0 0 0 0 0 0 0 0 0 0 0 0 0 0 0 0 0 0 0 0 0 0 0 0 0 0 0 0 0 0 0 0 0 0 0 0 0 0 0 0 0 0 0 0 0 0 0 0 0 0 0 0 0 0 0 0 0 0 0 0 0 0 0 0 0 0 0 0 0 0 0 0 0 0 0 0 0 0 0] % Parameter assumed  dAHvec=[0 -0.472 -0.944 -1.416 -1.889 -2.306 -2.716 -3.125 -3.535 -3.944 -4.342 -4.723 -5.104 -5.485 -5.867 -6.248 -6.629 -6.972 -7.314 -7.656 -7.997 -8.339 -8.681 -9.022 -9.457 -9.923 -10.389 -10.855 -11.321 -11.787 -12.254 -12.72 -13.106 -13.491 -13.876 -14.262 -14.647 -15.032 -15.417 -15.837 -16.264 -16.69 -17.116 -17.542 -17.987 -18.438 -18.889 -19.341 -19.792 -20.243 -20.694 -21.177 -21.71 -22.243 -22.776 -23.309 -23.842 -24.376 -24.909 -25.442 -25.915 -26.366 -26.816 -27.266 -27.717 -28.167 -28.617 -29.068 -29.518 -29.968 -30.419 -30.869 -31.319 -31.858 -32.41 -32.961 -33.512 -34.063 -34.615 -35.166 -35.717 -36.269 -36.802 -37.314 -37.826 -38.339 -38.851 -39.363 -39.875 -40.388 -40.9 -41.603 -42.38 -43.158 -43.935 -44.712 -45.49 -46.267 -47.044 -47.822] % Datasheet derived  dRleakvec=[0, 0, 0, 0] % Parameter not set  dR1vec=[0, 0, 0, 0] % Parameter not set  dR2vec=[0, 0, 0, 0] % Parameter not set  dR3vec=[0, 0, 0, 0] % Parameter not set  dR4vec=[0, 0, 0, 0] % Parameter not set  dR5vec=[0, 0, 0, 0] % Parameter not set  dV0mat=[0, 0; 0, 0; 0, 0; 0, 0] % Parameter not set  dR0mat=[0, 0; 0, 0; 0, 0; 0, 0] % Parameter not set  dAHmat=[0, 0; 0, 0; 0, 0; 0, 0] % Parameter not set  dRleakmat=[0, 0; 0, 0; 0, 0; 0, 0] % Parameter not set  dR1mat=[0, 0; 0, 0; 0, 0; 0, 0] % Parameter not set  dR2mat=[0, 0; 0, 0; 0, 0; 0, 0] % Parameter not set  dR3mat=[0, 0; 0, 0; 0, 0; 0, 0] % Parameter not set  dR4mat=[0, 0; 0, 0; 0, 0; 0, 0] % Parameter not set  dR5mat=[0, 0; 0, 0; 0, 0; 0, 0] % Parameter not set  prm_age_modeling=simscape.enum.tablebattery.prm_age_modeling.equation  storage_dt_age_vec=[0] % Parameter not set d  storage_T_age_vec=[273] % Parameter not set K  prm_age_OCV=simscape.enum.tablebattery.prm_age_OCV.OCV  OCV_age=0.9 % Parameter not set  SOC_age=0.6 % Parameter not set  prm_age_resistance=simscape.enum.tablebattery.prm_age.disabled  OCV_scaling_age_resistance=2.2134e6 % Parameter not set  OCV_offset_age_resistance=1.632e6 % Parameter not set  temp_exp_age_resistance=0.515833569 % Parameter not set V  t_exp_age_resistance=0.75 % Parameter not set  T_age_vec_resistance=[273.15, 298.15, 323.15] % Parameter not set K  dt_age_vec_resistance=[0, 90, 180, 270] % Parameter not set d  dR0_age_vec=[0, 0, 0] % Parameter not set  t_meas_dR0_age=100 % Parameter not set d  dR0_age_mat=[0, 0, 0; 0, 0, 0; 0, 0, 0; 0, 0, 0] % Parameter not set  prm_age_capacity=simscape.enum.tablebattery.prm_age.disabled  OCV_scaling_age_capacity=1.5097e07 % Parameter not set  OCV_offset_age_capacity=8.3625e06 % Parameter not set  temp_exp_age_capacity=0.6011 % Parameter not set V  t_exp_age_capacity=0.75 % Parameter not set  T_age_vec_capacity=[273.15, 298.15, 323.15] % Parameter not set K  dt_age_vec_capacity=[0, 90, 180, 270] % Parameter not set d  dAH_age_vec=[0, 0, 0] % Parameter not set  t_meas_dAH_age=100 % Parameter not set d  dAH_age_mat=[0, 0, 0; 0, 0, 0; 0, 0, 0; 0, 0, 0] % Parameter not set  thermal_port=simscape.enum.thermaleffects.omit  temperature=298.15 % Parameter not set K  thermal_mass=14670 % Parameter assumed J/K  i_specify=off  i_priority=None  i=0 A  i_nominal_specify=off  i_nominal_value=1  i_nominal_unit=A  v_specify=off  v_priority=None  v=0 V  v_nominal_specify=off  v_nominal_value=1  v_nominal_unit=V  stateOfCharge_specify=on  stateOfCharge_priority=High  stateOfCharge=0.2  stateOfCharge_nominal_specify=off  stateOfCharge_nominal_value=1  stateOfCharge_nominal_unit=1  num_cycles_specify=off  num_cycles_priority=High  num_cycles=0  num_cycles_nominal_specify=off  num_cycles_nominal_value=1  num_cycles_nominal_unit=1  cell_temperature_specify=off  cell_temperature_priority=High  cell_temperature=298.15 K  cell_temperature_nominal_specify=off  cell_temperature_nominal_value=1  cell_temperature_nominal_unit=K
      settings: AttributesFormatString=Valence:U24_24XP  InternalSimscapePortConfiguration="{\"Bottom\":[],\"Left\":[{\"id\":\"p\",\"label\":\"+\",\"type\":\"foundation.electrical.electrical\"},{\"id\":\"soc\",\"label\":\"SOC\",\"type\":\"output\"}],\"Right\":[{\"id\":\"n\",\"label\":\"-\",\"type\":\"foundation.electrical.electrical\"}],\"Top\":[]}"
      settings: LibrarySourceBlock=|
      | batt_lib/Cells/Battery
      | (Table-Based)
  Boost Converter : Subsystem  VariantControl=boostCircuit == 1
  Capacitor : fl_lib/Electrical/Electrical Elements/Capacitor  c=boost.inputCapacitor F  r=1e-6 Ohm  g=0 1/Ohm  i_specify=off  i_priority=None  i=0 A  i_nominal_specify=off  i_nominal_value=1  i_nominal_unit=A  v_specify=off  v_priority=None  v=solarPlant.startMPPTValue V  v_nominal_specify=off  v_nominal_value=1  v_nominal_unit=V  vc_specify=on  vc_priority=High  vc=solarPlant.startMPPTValue V  vc_nominal_specify=off  vc_nominal_value=1  vc_nominal_unit=V
  DC Current Sensor : Subsystem
      mask Display: disp('i')
  DC Output Voltage Sensor : Subsystem
      mask Display: disp('v')
  DC Voltage Sensor : Subsystem
      mask Display: disp('v');
  Electrical Reference : fl_lib/Electrical/Electrical Elements/Electrical Reference
  Gain : Gain  Gain=1e-3
  Gain1 : Gain  Gain=0.5
  Irradiance : Subsystem
  Monitoring : Subsystem
  PS-Simulink Converter : nesl_utility/PS-Simulink Converter  PhysicalDomain=network_engine_domain  SubClassName=ps_output  LeftPortType=input  RightPortType=output  PseudoPeriodic=off  Frequencies=[]  VectorFormat=inherit  Unit=inherit  AffineConversion=off
  PS-Simulink Converter1 : nesl_utility/PS-Simulink Converter  PhysicalDomain=network_engine_domain  SubClassName=ps_output  LeftPortType=input  RightPortType=output  PseudoPeriodic=off  Frequencies=[]  VectorFormat=inherit  Unit=inherit  AffineConversion=off
  PV Control : Subsystem
  Product : Product
  Scope : Scope  NumInputPorts=4
      settings: TimeSpan=t_sim2(end)  ActiveDisplayYMinimum=-6.6358431922855825  ActiveDisplayYMaximum=59.722588730570259
  Scope1 : Scope
      settings: ActiveDisplayYMinimum=0.14517600353103338  ActiveDisplayYMaximum=0.69293859438410943  DataLoggingVariableName=SOC  DataLoggingSaveFormat=Structure
  Simulink-PS Converter : nesl_utility/Simulink-PS Converter  PhysicalDomain=network_engine_domain  SubClassName=ps_input  LeftPortType=input  RightPortType=output  PseudoPeriodic=off  Frequencies=[]  NoiseDistribution=none  NoiseParameters=[]  Unit=1  AffineConversion=off  FilteringAndDerivatives=provide  SimscapeFilterOrder=1  InputFilterTimeConstant=0.001  UdotUserProvided=0
  Slider Switch : SliderSwitchBlock
  Solar PV Power kW1 : DisplayBlock  Transparency=1  GridColor=[0.502, 0.502, 0.502]
  Solar PV Power kW2 : DisplayBlock  Transparency=1  GridColor=[0.502, 0.502, 0.502]
  Solar PV Power kW3 : DisplayBlock  Transparency=1  GridColor=[0.502, 0.502, 0.502]
  Solar Plant : Subsystem
  Solver Configuration : nesl_utility/Solver Configuration  PhysicalDomain=network_engine_domain  SubClassName=solver  LeftPortType=input  RightPortType=generic  Tones=[]  Harmonics=[]  SimulateNoise=off  Profile=off  UseLocalSampling=off  EnableSwitchedLinearOptims=on  FrequencyDomain=off  UseCCode=off  RelTol=0.001  AbsTol=1e-06  MinStep=1e-09  ToWorkspace=off  RevertToSquareIcSolve=off  NumHomotopyIterations=100  PhasorMode=off  PhasorModeNumHarmonics=1  ConsistencySolver=NEWTON_FTOL  IndexReductionMethod=DerivativeReplacement  DoDC=off  ResidualTolerance=1e-9  ConsistencyTolSource=GLOBAL  ConsistencyAbsTol=0.001  ConsistencyRelTol=0.001  ConsistencyTolFactor=0.001  UseLocalSolver=off  LocalSolverChoice=NE_BACKWARD_EULER_ADVANCER  ResolveIndetEquations=on  FunctionEvalNumThread=1  LocalSolverSampleTime=1e-6  DoFixedCost=off  MaxNonlinIter=10  MaxModeIter=2  ComputeImpulses=off  ImpulseIterations=2  LinearAlgebra=auto  LinearAlgebraNumThread=0  EquationFormulation=NE_TIME_EF  DelaysMemoryBudget=1024  AutomaticFiltering=on  FilteringTimeConstant=0.001  PartitionStorageMethod=AS_NEEDED  PartitionMemoryBudget=1024  PartitionMethod=FAST  MultibodyUseLocalSolver=off  MultibodyLocalSolverChoice=ODE1  MultibodyLocalSolverSampleTime=0.001
  tag scope: Gpv=global
  wires:
  PV Control/1(Gate) -> [Gpv]
  [Vo] -> Scope/1  "DC Bus Voltage Vo (V)"
  Irradiance/1(Irad) -> Simulink-PS Converter/1
  [Vpv] -> Product/2, Scope/3  "Solar Panel Voltage Vpv (V)"
  [Gpv] -> Boost Converter/1(m)
  [Vo] -> PV Control/1(Vo)
  [Ipv] -> Product/1, Scope/2  "Solar PV Current Ipv (A)"
  Product/1 -> Gain/1  "Solar Power(W)"
  Gain/1 -> Scope/4  "Solar Power (kW)"
  [Ipv] -> PV Control/2(Ipv)
  [Vpv] -> PV Control/3(Vpv)
  [IL] -> PV Control/4(IL)
  PS-Simulink Converter/1 -> Add/1
  PS-Simulink Converter1/1 -> Add/2
  Add/1 -> Gain1/1
  Gain1/1 -> Scope1/1  "SOC"
  connections:
  Boost Converter/RConn2 -- Battery (Table-Based)1/RConn1 -- DC Output Voltage Sensor/LConn1
  Solar Plant/RConn2 -- Solver Configuration/RConn1 -- Electrical Reference/LConn1 -- Boost Converter/LConn2 -- DC Voltage Sensor/LConn1 -- Capacitor/RConn1
  DC Voltage Sensor/RConn1 -- DC Current Sensor/LConn1 -- Capacitor/LConn1 -- Boost Converter/LConn1
  DC Output Voltage Sensor/RConn1 -- AC Current Sensor2/RConn1 -- Boost Converter/RConn1
  Simulink-PS Converter/RConn1 -- Solar Plant/LConn1
  DC Current Sensor/RConn1 -- Solar Plant/RConn1
  Battery (Table-Based)1/LConn1 -- Battery (Table-Based)/RConn1
  AC Current Sensor2/LConn1 -- Battery (Table-Based)/LConn1
  Battery (Table-Based)/LConn2 -- PS-Simulink Converter/LConn1
  PS-Simulink Converter1/LConn1 -- Battery (Table-Based)1/LConn2
